simulink model "flightControlSystem"  (R2021a)
settings: Solver=ode3  StartTime=0  StopTime=TFinal  FixedStep=Ts  RelTol=1e-3  EnableMultiTasking=on
undefined symbols (not defined in the file): codertarget, Controller, DiscIntNeverNeededParam, Discrete, Estimator, g, init, Sensors, Time, Ts, var_acc_angle_N, var_bias_gyr_N, var_gyro_p_N, Vehicle
libraries: simulink x38, pid_lib x4, ctrlSharedLib x4, sharedtransform x3, parrotlib x1
(part 3 of 3)

== stateflow chart flightControlSystem/Control System/Path Planning/Chart ==
  state Stage_1
    state Initial_
      entry:
      during:
    state Stage1
      entry:
      zValue=-1.1;
      dir_=dirInput;
      during:
      [coneSumVal,vidOut]=coneSum(dir_,coneCoords,filteredImage)
      xValue=0;yValue=0;
      dirOut=0;stageOut=0;
    (default) -> Initial_
    Initial_ -> Stage1 : [stage==0]
  state Stage_3_
    entry:
    during:
    state EndTrackCircleApproach
    state CircleCentringAndDescend
    state initial_
      entry:
      during:
    (default) -> initial_
    initial_ -> EndTrackCircleApproach
    EndTrackCircleApproach -> CircleCentringAndDescend
  state Stage_2_
    state StraightPath_
      entry:
      dir_=dirInput;
      [coneSumVal,vidOut]=coneSum(dir_,coneCoords,filteredImage);
      during:
      [coneSumVal,vidOut]=coneSum(dir_,coneCoords,filteredImage);
      if coneSumVal>420
      a=0.1;
      xValue=a*cos(dir_);
      yValue=a*sin(dir_);
      genDir=genDirection(dir_)
      dirOut=dir_;
      end
    state trackEndCheck_
      entry:
      turnCheck=0;
      [trackEndFalseSum,notUsed]=coneSum(dir_,trackEndFalse,filteredImage);
      if (trackEndFalseSum) <52
      [trackEndTrueSum,notUsed]=coneSum(dir_,trackEndTrue,filteredImage);
      if (trackEndTrueSum)>100
      trackEndCheck=1;
      stageOut=3;
      else
      turnCheck=1;
      end
      else
      turnCheck=1;
      end
      dirOut=dir_;
      during:
    state Turning_
      entry:
      straightPathCheck=0;
      during:
      dirOld=dir_;
      dirNew  = turnScan(filteredImage,coneCoords, dirOld);
      if abs(dirNew-dirOld)<(0.1*dirOld)
      %will turn back
      else
      dir_=dirNew;
      straightPathCheck=1;
      dirOut=dir_;
      end
      dirOut=dir_;
    (default) -> StraightPath_
    StraightPath_ -> trackEndCheck_ : [coneSumVal<420]
    trackEndCheck_ -> Turning_ : [turnCheck>0]
    Turning_ -> StraightPath_ : [straightPathCheck==1]
  state trackEndCricleApproach_ [commented out]
    entry:
    during:
    [ctrls_,check_] = trackEndDroneEnteringCircle(trackEndFalse,filteredImage,dir)
    xValue_=ctrls_(1);yValue_=ctrls_(2);
    circleApproachCheck_=check_;
  state Stage 3: [commented out]
    state Scan1_ [commented out]
      entry:
      during:
      [ctrls,check] = trackEndDroneEnteringCircle(trackEndFalse,filteredImage,dir)
      xValue=ctrls(1);yValue=ctrls(2);
      circleApproachCheck=check
    state Scan2 [commented out]
    (default) -> Scan1_ [commented out]
  (default) -> Stage_1
  Stage_1 -> Stage_3_ [order 1] : [stage==3]
  Stage_1 -> Stage_2_ [order 2] : [zValueRef<-1.05 && zValueRef>-1.2 && sum(coneSumVal,"all")>50]
  data: dir1 function_input; coneCoords1 function_input; filteredImage1 function_input; sumVal function_output; video function_output; filteredImage2 function_input; coneCoords2 function_input; dirOld2 function_input; dirNew2 function_output; dir function_input; output function_output; zValueRef input; coneCoords input; filteredImage input size=[120,160]; trackEndFalse input size=[2,919]; trackEndTrue input size=[2,919]; trackEndTrueSum local size=1; zValue output; coneSumVal local size=1; turnCheck local size=1; trackEndFalseSum local size=1; xValue output; yValue output; dirOut output size=1; dirInput input; dir_ local size=1; dirNew local size=1; dirOld local size=1; straightPathCheck local size=1; coneSumValCurr local size=1; stage input; a local size=1; stageOut output size=1; trackEndCheck local; vidOut output; notUsed local; genDir output
  function [sumVal,video] = coneSum(dir1,coneCoords1,filteredImage1):
    | function [sumVal,video] = coneSum(dir1,coneCoords1,filteredImage1)
    | %check =1 if on straight path
    | 
    | %% transform/rotate the cone
    | trpseMatrix=[cos(dir1), sin(dir1) ; -sin(dir1), cos(dir1)];
    | 
    | A=trpseMatrix*coneCoords1; %cone points in direction, dir
    | 
    | x_range = round(A(1,:));
    | y_range = round(A(2,:));
    | 
    | %% centres the cone
    | [mx, my]=size(filteredImage1);
    | 
    | mx_c=round(mx/2); my_c=round(my/2);
    | mx_range = x_range +  mx_c;
    | my_range = my_c - y_range; %cone has been placed in the middle
    | 
    | 
    | %% identifies pixels that are on path and in the rotating cone
    | 
    | screen=zeros(size(filteredImage1));
    | 
    | for i = 1:length(my_range)
    |     if my_range(i)==-11||mx_range(i)==-11
    |     fprintf("")
    |     
    |     
    |     end
    |     screen(my_range(i),mx_range(i)) = filteredImage1(my_range(i),mx_range(i));
    | end
    | 
    | %% summation
    | 
    | sumVal=sum(screen,'all')/255;
    | video=screen;
    | 
    | end
  function dirNew2  = turnScan(filteredImage2,coneCoords2, dirOld2):
    | function dirNew2  = turnScan(filteredImage2,coneCoords2, dirOld2)
    | dirNew2=0;
    | 
    | turningCheck=0;
    | phi=pi()/6;
    | dir=dirOld2;
    | thetaRange=zeros(1,11);
    | count=2;
    | 
    | while ~turningCheck
    |     %iter 1
    |     sumValArray1=zeros(1,11);
    |     
    |     sumVal=coneSum(dir,coneCoords2,filteredImage2);
    |     sumValArray1(1)=sumVal;
    |     
    |     thetaRange(1)=dir;
    |     
    |     iter1=1;
    |     i=2;
    |     
    |     dirCurPlus=0;
    |     dirCurMinus=0;
    |     
    |     while iter1<count
    |         dirCurPlus=dirCurPlus+phi;
    |         dirCurMinus=dirCurMinus-phi;
    |         
    |         thetaRange(i)=dirCurPlus;
    |         thetaRange(i+1)=dirCurMinus;
    |         
    |          sumValPlus=coneSum(dirCurPlus,coneCoords2,filteredImage2);
    |          sumValMinus=coneSum(dirCurMinus,coneCoords2,filteredImage2);
    |          
    |         sumValArray1(i)=sumValPlus;
    |         sumValArray1(i+1)=sumValMinus;
    |         
    |         i=i+2;
    |         iter1=iter1+1;
    |     end
    |     
    |     [val pos]=max(sumValArray1);
    |     
    |     dir1=thetaRange(pos);
    |     
    |     
    |        %iter 2
    |        
    |     dir=dir1;
    |     
    |     sumValArray2=zeros(1,11);
    |     sumVal2=coneSum(dir,coneCoords2,filteredImage2);
    |     sumValArray2(1)=sumVal2;
    |     
    |     thetaRange2=zeros(1,11);
    |     thetaRange2(1)=dir;
    |     
    |     iter=1;
    |     i=2;
    |     
    |     dirCurPlus=0;
    |     dirCurMinus=0;
    |     
    |     while iter<count
    |         dirCurPlus=dirCurPlus+phi;
    |         dirCurMinus=dirCurMinus-phi;
    |         
    |         thetaRange2(i)=dirCurPlus;
    |         thetaRange2(i+1)=dirCurMinus;
    |         
    |          sumValPlus=coneSum(dirCurPlus,coneCoords2,filteredImage2);
    |          sumValMinus=coneSum(dirCurMinus,coneCoords2,filteredImage2);
    |          
    |         sumValArray2(i)=sumValPlus;
    |         sumValArray2(i+1)=sumValMinus;
    |         
    |         i=i+2;
    |         iter=iter+1;
    |     end
    |     
    |     [val pos]=max(sumValArray2);
    |     
    |     dir2=thetaRange2(pos);
    |     
    |     %check
    |     
    |     if abs(dir1-dir2)<0.1*dir2
    |         turningCheck=1;
    |         dirNew2=(dir1+dir2)/2;
    |     elseif count==5
    |             turningCheck=1;
    |             dirNew2=0;
    | %             error("cant find!!!!")
    |     else
    |         count=count+1;
    |         turningCheck=0;
    |     end
    | 
    | end
    |    
    | 
    | end
  function output =genDirection(dir):
    | function output =genDirection(dir)
    | if dir>7/4*pi || dir<pi/4
    |     output=5;
    | elseif dir>pi/4&&dir<3/4*pi
    |     output=1;
    | elseif dir>3/4*pi &&dir<5/4*pi
    |     output=4;
    | elseif dir>5/4*pi&&dir<7/4*pi
    |     output=2;
    | else
    |     output=1000000000;
    | end

== matlab function flightControlSystem/Control System/Path Planning/MATLAB Function1 ==
  data: h input; coneCoords output; increment input
function coneCoords  = coneCreate(h,increment)
%[S] = coneCreate(50,1)
% y_range = 0:h; %height

% pre allocating a matrix for the cone x and y coordinate positions
coneCoordsCur = ones(919, 2);

% counters
m=1;
c=1; % used to reference spots within matrix S, used to store values of the cone.
n=1; %used to determine the range of x in each lattice of the cone %used to determine the increase in x range as you jump from lattice to lattice

for y = 0:h
    
    for x = -n:n

        coneCoordsCur(c,1) = x;
        coneCoordsCur(c,2) = y;
        c=c+1;
    end
    %this line is used to indirectly adjust the cone angle, the larger the
    %increment to m, the larger the cone value as it lenghtens the range of
    %rows each layer of the cone. imagine the cone as being built from the
    %point at the origin to the widest part in the positive y direction
    m = m+increment;
    n=round(m);
end
    
%% centering the cone
% [my,mx] = size(filteredImage);
% 
% % we have created the cone in the cartesian reference with 0,0 origin
% % reference, however matlab matrices start indices at 1,1 at the top left
% % increasing towards bottom right. hence to adjust, we must find the
% % relative centre of the image matrix
% 
% mx_c = round(0.5*mx);
% my_c = round(0.5*my);   


%% centring and creating the cone
coneCoordsCur = coneCoordsCur'; % from [x y] --> [x;y]

% x_range = coneCoordsCur(1,:);
% y_range = coneCoordsCur(2,:);
% 
% mx_range = x_range +  mx_c;
% % my_range = my_c - y_range;
% 
% coneCoords=[mx_range;my_range];

coneCoords=coneCoordsCur;

 
end

== matlab function flightControlSystem/Control System/Path Planning/MATLAB Function2 ==
  data: yh input; trackEndTrue output; coneCoords input; trackEndFalse output
function [trackEndTrue,trackEndFalse] = trackEndDetectFilterCreate(yh,coneCoords)
%S=[x; y] %%check for this!!!
sections=3;
yrange=linspace(0,yh,sections+1);

trackEndTrue=zeros(2, length(coneCoords));
trackEndFalse=zeros(2, length(coneCoords));

x=coneCoords(1,:);
y=coneCoords(2,:);

for i=1:length(coneCoords)
    if y(i)>round(yrange(end-1))
        trackEndTrue(1,i)=x(i);
        trackEndTrue(2,i)=y(i);
    end
    
    if round(yrange(3))> y(i) && y(i)>round(yrange(2))
            trackEndFalse(1,i)=x(i);
            trackEndFalse(2,i)=y(i);
    end
end
